simulink model "goPtByAcf"  (Simulink 7.2)
settings: Solver=FixedStepDiscrete  SolverMode=MultiTasking  StartTime=0.0  StopTime=10.0  RelTol=1e-3
undefined symbols (not defined in the file or in its folder): get
libraries: dspstat3 x2, dspbuff3 x2, dspsnks4 x2, dspsrcs4 x1
settings Model: Creator=jang  LastModifiedBy=jang

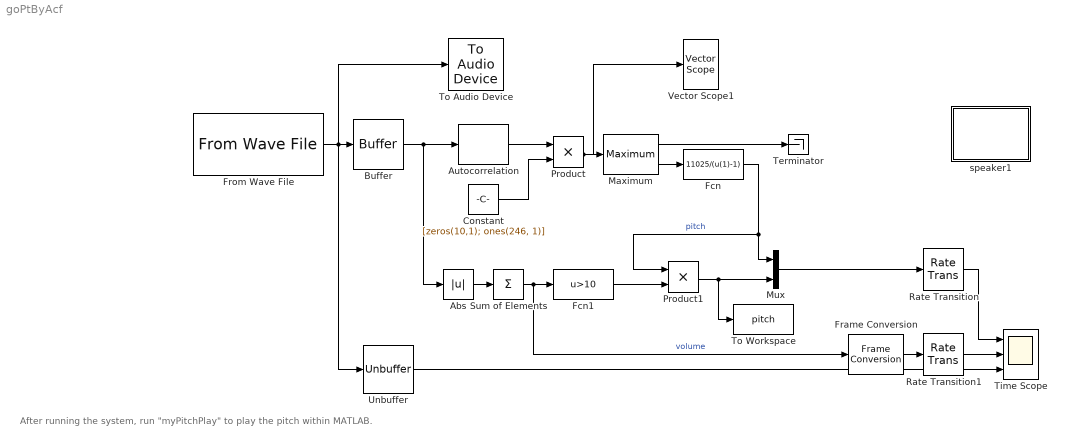
== system goPtByAcf ==
  note: After running the system, run "myPitchPlay" to play the pitch within MATLAB.
  Abs : Abs  OutDataType=sfix(16)  OutScaling=2^0
  Autocorrelation : dspstat3/Autocorrelation  DialogController=dspDDGCreate  DialogControllerArgs=DataTag0  AllPositiveLags=on  maxlag=1  bias=None  domain=Time  roundingMode=Floor  overflowMode=off
  Buffer : dspbuff3/Buffer  N=256  V=0  ic=0
  Constant : Constant  Value=[zeros(10,1); ones(246, 1)]  VectorParams1D=off  OutDataType=sfix(16)  OutScaling=2^0
      settings: SamplingMode=Frame based
  Fcn : Fcn  Expr=11025/(u(1)-1)
  Fcn1 : Fcn  Expr=u>10
  Frame Conversion : FrameConversion  OutFrame=Sample-based
  From Wave File : dspsrcs4/From Wave File  FileName=doremi.wav  SamplesPerFrame=256  MinBufSize=256  dType=double  bLoop=off  timesToPlay=1  restartMode=immediately after last sample  firstSampleOutput=off  lastSampleOutput=off
  Maximum : dspstat3/Maximum  DialogController=dspfixptddg.MinMax  DialogControllerArgs=DataTag1  fcn=Value and Index  reset=None  indexBase=One  operateOver=Each column  Dimension=1  colComp=on  operation=maximum  roiEnable=off  roiType=Rectangles  roiPortion=Entire ROI  roiOutput=Individual statistics for each ROI  roiFlag=off  roundingMode=Floor  overflowMode=off
  Mux : Mux  Inputs=2
  Product : Product  OutDataType=sfix(16)  OutScaling=2^0  RndMeth=Zero
  Product1 : Product  OutDataType=sfix(16)  OutScaling=2^0  RndMeth=Zero
  Rate Transition : RateTransition
  Rate Transition1 : RateTransition
  Sum of Elements : Sum  Inputs=+  OutDataType=sfix(16)  OutScaling=2^-10
  Terminator : Terminator
  Time Scope : Scope  NumInputPorts=3
      settings: TickLabels=on  TimeRange=10  YMin=0~0~-1  YMax=1200~100~1  DataFormat=Structure  MaxDataPoints=150000
  To Audio Device : dspsnks4/To Audio Device  DialogController=dspDDGCreate  DialogControllerArgs=DataTag2  deviceName=Default  inheritSampleRate=on  sampleRate=44100  deviceDatatype=Determine from input data type  autoBufferSize=on  bufferSize=4096  queueDuration=1.0
  To Workspace : ToWorkspace  VariableName=pitch  SampleTime=-1  SaveFormat=Structure
  Unbuffer : dspbuff3/Unbuffer  ic=0
  Vector Scope1 : dspsnks4/Vector Scope  DialogController=dspdialog.VectorScope  DialogControllerArgs=DataTag3  ScopeProperties=on  Domain=Time  HorizSpan=1  DisplayProperties=off  AxisGrid=on  Memory=off  FrameNumber=on  AxisLegend=on  AxisZoom=off  OpenScopeAtSimStart=on  OpenScopeImmediately=off  FigPos=get(0,'defaultfigureposition')  AxisProperties=off  XUnits=Hertz  XRange=[0...Fs/2]  InheritXIncr=on  XIncr=1  XLabel=Time  XLimit=Auto  XMin=0  XMax=1  XStart=0  YUnits=dB  YLabel=Amplitude  LineProperties=off
      settings: YMin=-5.31059112548828  YMax=8.44944610595703
  speaker1 : Subsystem
      settings: OpenFcn=myPitchPlay
      mask Display: disp('Play pitch\nheard\nby computer')
  wires:
  Abs/1 -> Sum of Elements/1
  Product/1 -> Maximum/1, Vector Scope1/1
  Maximum/2 -> Fcn/1
  Fcn/1 -> Product1/1, Mux/1  "pitch"
  Sum of Elements/1 -> Fcn1/1, Frame Conversion/1  "volume"
  Fcn1/1 -> Product1/2
  Product1/1 -> Mux/2, To Workspace/1
  Buffer/1 -> Autocorrelation/1, Abs/1
  Mux/1 -> Rate Transition/1
  From Wave File/1 -> To Audio Device/1, Unbuffer/1, Buffer/1
  Autocorrelation/1 -> Product/1
  Constant/1 -> Product/2
  Maximum/1 -> Terminator/1
  Unbuffer/1 -> Time Scope/3
  Rate Transition1/1 -> Time Scope/2
  Rate Transition/1 -> Time Scope/1
  Frame Conversion/1 -> Rate Transition1/1

== system goPtByAcf/speaker1 ==
